simulink model "controller_v12"  (R2022a)
settings: Solver=FixedStepDiscrete  StartTime=0.0  StopTime=inf  RelTol=1e-3
undefined symbols (not defined in the file): ctr, DiscIntNeverNeededParam, flt, IO397, mdl, rbt, rsim, som, ukf_P0_flat, ukf_prediction_time, ukf_s0, ukf_sys, ukf_use_prediction
libraries: simulink x31, slrealtimeloglib x14, slrealtimetgmanagement x5, slrealtimeseriallib x5, speedgoatlib_fpga_analog_io x4, speedgoatlib_fpga x2, speedgoatlib_fpga_dio x1, slrealtimeutilitieslib x1
(part 2 of 4)

== system controller_v12/Force//Torque to Trajectory Specs/force//torque to module thrust ==
  note: No YAW torque control at the moment
  thrust : Inport
  x Tq : Inport  Port=2
  y Tq : Inport  Port=3
  z Tq : Inport  Port=4
  Inputs : slrealtimeloglib/File Log  Commented=on  decimation=1
      settings: SourceProductBaseCode=XP
  Mux : Mux
  SaturatingRamp : DiscreteIntegrator  gainval=1  SampleTime=-1  UpperSaturationLimit=1  LowerSaturationLimit=0  ICPrevOutput=DiscIntNeverNeededParam  ICPrevScaledInput=DiscIntNeverNeededParam
  constant : Constant
  mapping scheme (flipping compataible) : MATLAB Function  TreatAsAtomicUnit=on  SystemSampleTime=mdl.T
  module thrusts (1-4) : Outport  PortDimensions=4
  wires:
  thrust/1 -> Mux/1
  x Tq/1 -> Mux/2
  y Tq/1 -> Mux/3
  z Tq/1 -> Mux/4
  Mux/1 -> Inputs/1, mapping scheme (flipping compataible)/2(inputs)
  mapping scheme (flipping compataible)/1(module_f) -> module thrusts (1-4)/1
  constant/1 -> SaturatingRamp/1
  SaturatingRamp/1 -> mapping scheme (flipping compataible)/1(time)

== system controller_v12/Force//Torque to Trajectory Specs/nominal desired voltage ==
  Force : Inport
  Forces : slrealtimeloglib/File Log  Commented=on  decimation=1  inputProcessing=Elements as channels (sample based)
      settings: SourceProductBaseCode=XP
  SaturatingRamp : DiscreteIntegrator  gainval=1  SampleTime=-1  UpperSaturationLimit=1  LowerSaturationLimit=0  ICPrevOutput=DiscIntNeverNeededParam  ICPrevScaledInput=DiscIntNeverNeededParam
  Switch : Switch  Criteria=u2 > Threshold  SaturateOnIntegerOverflow=off  InputSameDT=off
  constant1 : Constant
  "force to voltage (hovering) " : Subsystem
  force to voltage flipping : Subsystem
  map_selection : MATLAB Function  TreatAsAtomicUnit=on  SystemSampleTime=mdl.T
  Voltages : Outport
  wires:
  Force/1 -> Forces/1, force to voltage flipping/1(force), "force to voltage (hovering) "/1(force)
  "force to voltage (hovering) "/1(Vout) -> Switch/1
  force to voltage flipping/1(Vout) -> Switch/3
  Switch/1 -> Voltages/1
  map_selection/1(hover_map) -> Switch/2
  constant1/1 -> SaturatingRamp/1
  SaturatingRamp/1 -> map_selection/1(time)

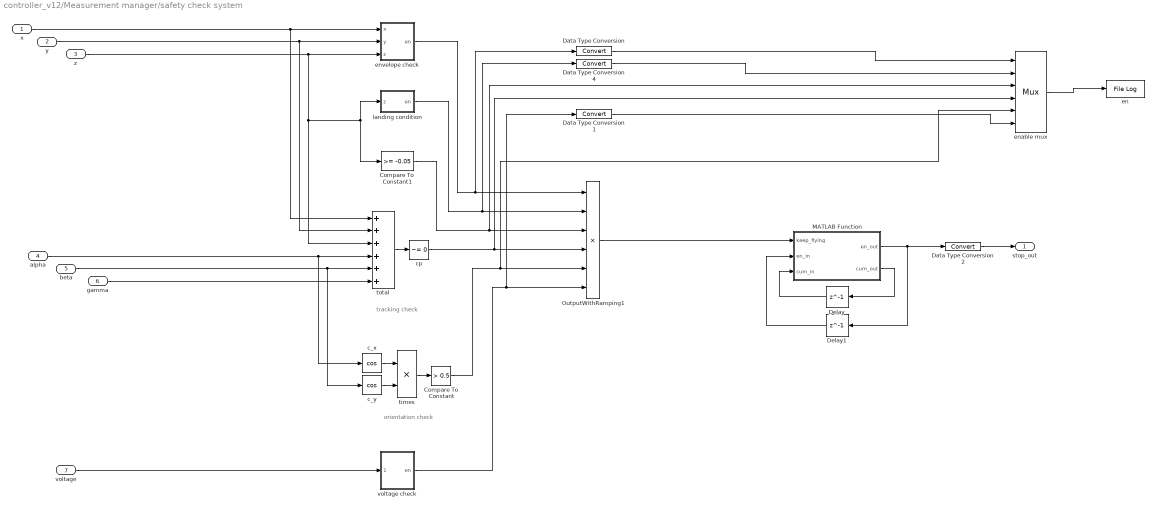
== system controller_v12/Measurement manager/safety check system ==
  note: orientation check
  note: tracking check
  x : Inport
  y : Inport  Port=2
  z : Inport  Port=3
  alpha : Inport  Port=4
  beta : Inport  Port=5
  gamma : Inport  Port=6
  voltage : Inport  Port=7
  Compare To Constant : simulink/Logic and Bit Operations/Compare To Constant  relop=>  const=0.5  OutDataTypeStr=uint8
  Compare To Constant1 : simulink/Logic and Bit Operations/Compare To Constant  relop=>=  const=-0.05  OutDataTypeStr=uint8
  Data Type Conversion{,1..2,4} (4 alike) : DataTypeConversion  SaturateOnIntegerOverflow=off  RndMeth=Floor
  Delay : Delay  DelayLength=1
  Delay1 : Delay  DelayLength=1  InitialCondition=1
  MATLAB Function : MATLAB Function  TreatAsAtomicUnit=on
  OutputWithRamping1 : Product  Inputs=6  RndMeth=Zero
  c_x : Trigonometry  Operator=cos
  c_y : Trigonometry  Operator=cos
  cp : simulink/Logic and Bit Operations/Compare To Zero  relop=~=  OutDataTypeStr=uint8
  en : slrealtimeloglib/File Log  decimation=1  inputProcessing=Elements as channels (sample based)
      settings: SourceProductBaseCode=XP
  enable mux : Mux  Inputs=6
      settings: DisplayOption=signals
  envelope check : MATLAB Function  TreatAsAtomicUnit=on
  landing condition : Subsystem
  times : Product  RndMeth=Zero
  total : Sum  Inputs=++++++
  voltage check : MATLAB Function  TreatAsAtomicUnit=on  SystemSampleTime=mdl.T
  stop_out : Outport
  wires:
  Compare To Constant1/1 -> enable mux/3, OutputWithRamping1/3
  y/1 -> envelope check/2(y), total/2
  cp/1 -> enable mux/4, OutputWithRamping1/4
  envelope check/1(en) -> Data Type Conversion/1, OutputWithRamping1/1
  enable mux/1 -> en/1
  landing condition/1(en) -> Data Type Conversion4/1, OutputWithRamping1/2
  Data Type Conversion/1 -> enable mux/1
  times/1 -> Compare To Constant/1
  voltage check/1(en) -> Data Type Conversion1/1, OutputWithRamping1/6
  z/1 -> total/3, Compare To Constant1/1, landing condition/1(z), envelope check/3(z)
  Compare To Constant/1 -> enable mux/5, OutputWithRamping1/5
  total/1 -> cp/1
  Data Type Conversion4/1 -> enable mux/2
  x/1 -> total/1, envelope check/1(x)
  alpha/1 -> total/4, c_x/1
  beta/1 -> total/5, c_y/1
  c_x/1 -> times/1
  c_y/1 -> times/2
  Data Type Conversion1/1 -> enable mux/6
  voltage/1 -> voltage check/1(voltage)
  gamma/1 -> total/6
  OutputWithRamping1/1 -> MATLAB Function/1(keep_flying)
  Delay1/1 -> MATLAB Function/2(en_in)
  MATLAB Function/1(en_out) -> Delay1/1, Data Type Conversion2/1
  Delay/1 -> MATLAB Function/3(cum_in)
  MATLAB Function/2(cum_out) -> Delay/1
  Data Type Conversion2/1 -> stop_out/1

== system controller_v12/Phantom trigger/timer1 ==
  SaturatingRamp : DiscreteIntegrator  gainval=1  SampleTime=-1  UpperSaturationLimit=1  LowerSaturationLimit=0  ICPrevOutput=DiscIntNeverNeededParam  ICPrevScaledInput=DiscIntNeverNeededParam
  constant : Constant
  time : Outport
  wires:
  constant/1 -> SaturatingRamp/1
  SaturatingRamp/1 -> time/1

== system controller_v12/closed loop en/safety1 ==
  In1 : Inport
  Compare To Constant1 : simulink/Logic and Bit Operations/Compare To Constant  relop=<=  const=inf  OutDataTypeStr=uint8
  Switch1 : Switch  Threshold=0.5  SaturateOnIntegerOverflow=off  InputSameDT=off
  zero1 : Constant  Value=0
  Out1 : Outport
  wires:
  In1/1 -> Switch1/1, Compare To Constant1/1
  Compare To Constant1/1 -> Switch1/2
  zero1/1 -> Switch1/3
  Switch1/1 -> Out1/1

== system controller_v12/closed loop en/safety2 ==
  In1 : Inport
  Compare To Constant1 : simulink/Logic and Bit Operations/Compare To Constant  relop=<=  const=inf  OutDataTypeStr=uint8
  Switch1 : Switch  Threshold=0.5  SaturateOnIntegerOverflow=off  InputSameDT=off
  zero1 : Constant  Value=0
  Out1 : Outport
  wires:
  In1/1 -> Switch1/1, Compare To Constant1/1
  Compare To Constant1/1 -> Switch1/2
  zero1/1 -> Switch1/3
  Switch1/1 -> Out1/1

== system controller_v12/closed loop en/safety3 ==
  In1 : Inport
  Compare To Constant1 : simulink/Logic and Bit Operations/Compare To Constant  relop=<=  const=inf  OutDataTypeStr=uint8
  Switch1 : Switch  Threshold=0.5  SaturateOnIntegerOverflow=off  InputSameDT=off
  zero1 : Constant  Value=0
  Out1 : Outport
  wires:
  In1/1 -> Switch1/1, Compare To Constant1/1
  Compare To Constant1/1 -> Switch1/2
  zero1/1 -> Switch1/3
  Switch1/1 -> Out1/1

== system controller_v12/closed loop en/safety4 ==
  In1 : Inport
  Compare To Constant1 : simulink/Logic and Bit Operations/Compare To Constant  relop=<=  const=inf  OutDataTypeStr=uint8
  Switch1 : Switch  Threshold=0.5  SaturateOnIntegerOverflow=off  InputSameDT=off
  zero1 : Constant  Value=0
  Out1 : Outport
  wires:
  In1/1 -> Switch1/1, Compare To Constant1/1
  Compare To Constant1/1 -> Switch1/2
  zero1/1 -> Switch1/3
  Switch1/1 -> Out1/1

== system controller_v12/signal generator/Bias_Signal ==
  note: time constant = 0.002sec
  QuasiEnable : Inport
  BiasVolts : Inport  Port=2
  AveragedBias : Subsystem
  PreGain : Gain
  Product : Product  RndMeth=Zero
  SIgnalForRamp_binary : Subsystem
  SaturatingRamp : DiscreteIntegrator  gainval=10  SampleTime=-1  LimitOutput=on  UpperSaturationLimit=1  LowerSaturationLimit=0  ICPrevOutput=DiscIntNeverNeededParam  ICPrevScaledInput=DiscIntNeverNeededParam
  BiasD2A : Outport
  wires:
  PreGain/1 -> BiasD2A/1
  BiasVolts/1 -> AveragedBias/1(In1)
  QuasiEnable/1 -> SIgnalForRamp_binary/1(In1)
  SIgnalForRamp_binary/1(Out1) -> SaturatingRamp/1
  SaturatingRamp/1 -> Product/1
  AveragedBias/1(Out1) -> Product/2
  Product/1 -> PreGain/1

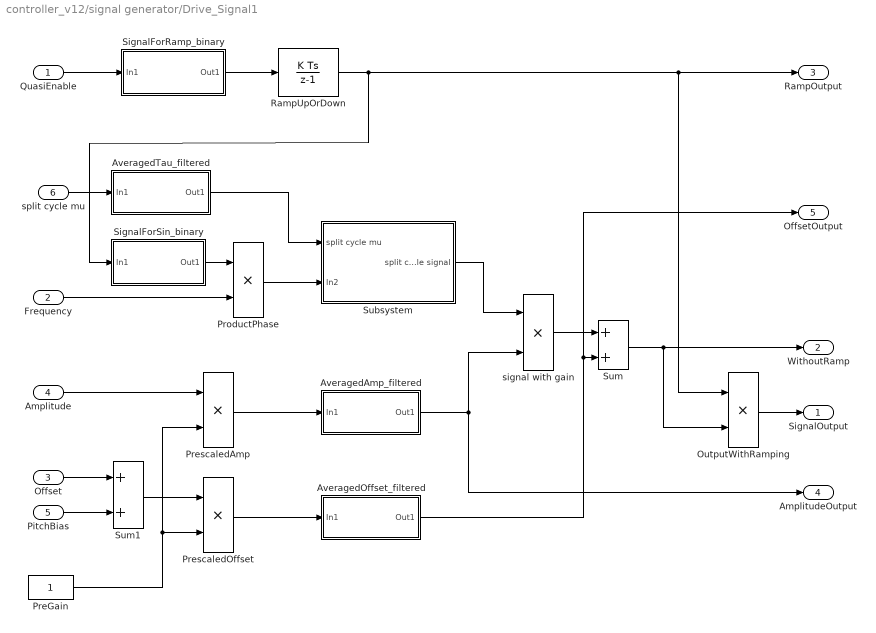
== system controller_v12/signal generator/Drive_Signal1 ==
  QuasiEnable : Inport
  Frequency : Inport  Port=2
  Offset : Inport  Port=3
  Amplitude : Inport  Port=4
  PitchBias : Inport  Port=5
  split cycle mu : Inport  Port=6
  AveragedAmp_filtered : Subsystem
  AveragedOffset_filtered : Subsystem
  AveragedTau_filtered : Subsystem
  OutputWithRamping : Product  RndMeth=Zero
  PreGain : Constant
  PrescaledAmp : Product  RndMeth=Zero
  PrescaledOffset : Product  RndMeth=Zero
  ProductPhase : Product  RndMeth=Zero
  RampUpOrDown : DiscreteIntegrator  gainval=10  SampleTime=-1  LimitOutput=on  UpperSaturationLimit=1  LowerSaturationLimit=0  ICPrevOutput=DiscIntNeverNeededParam  ICPrevScaledInput=DiscIntNeverNeededParam
  SignalForRamp_binary : Subsystem
  SignalForSin_binary : Subsystem
  Subsystem : Subsystem
  Sum : Sum
  Sum1 : Sum
  signal with gain : Product  RndMeth=Zero
  SignalOutput : Outport
  WithoutRamp : Outport  Port=2
  RampOutput : Outport  Port=3
  AmplitudeOutput : Outport  Port=4
  OffsetOutput : Outport  Port=5
  wires:
  PrescaledAmp/1 -> AveragedAmp_filtered/1(In1)
  Sum/1 -> OutputWithRamping/2, WithoutRamp/1
  RampUpOrDown/1 -> RampOutput/1, OutputWithRamping/1, SignalForSin_binary/1(In1)
  QuasiEnable/1 -> SignalForRamp_binary/1(In1)
  SignalForRamp_binary/1(Out1) -> RampUpOrDown/1
  Amplitude/1 -> PrescaledAmp/1
  signal with gain/1 -> Sum/1
  Frequency/1 -> ProductPhase/2
  SignalForSin_binary/1(Out1) -> ProductPhase/1
  ProductPhase/1 -> Subsystem/2(In2)
  AveragedOffset_filtered/1(Out1) -> Sum/2, OffsetOutput/1
  PrescaledOffset/1 -> AveragedOffset_filtered/1(In1)
  PreGain/1 -> PrescaledAmp/2, PrescaledOffset/2
  OutputWithRamping/1 -> SignalOutput/1
  AveragedAmp_filtered/1(Out1) -> signal with gain/2, AmplitudeOutput/1
  Sum1/1 -> PrescaledOffset/1
  Offset/1 -> Sum1/1
  PitchBias/1 -> Sum1/2
  AveragedTau_filtered/1(Out1) -> Subsystem/1(split cycle mu)
  split cycle mu/1 -> AveragedTau_filtered/1(In1)
  Subsystem/1(split cycle signal) -> signal with gain/1

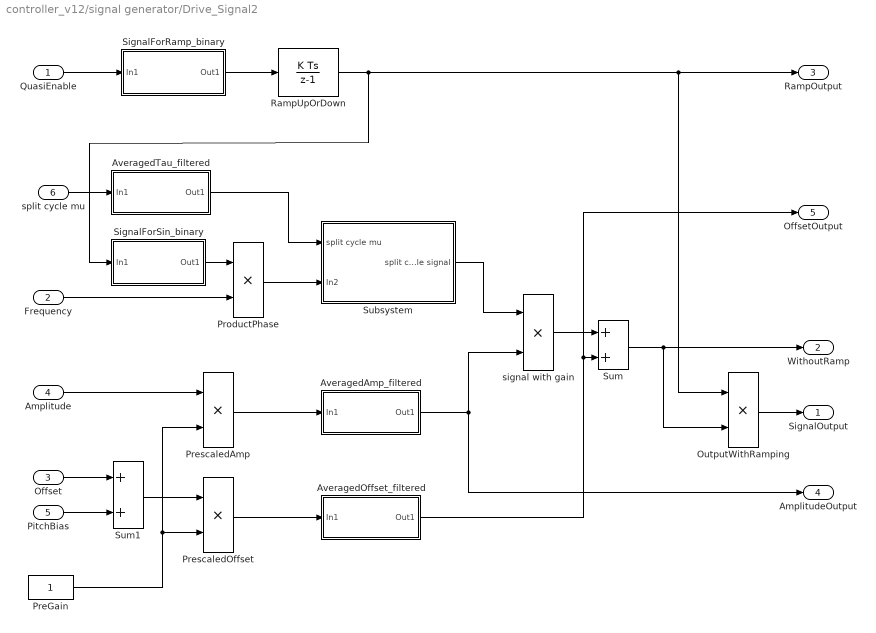
== system controller_v12/signal generator/Drive_Signal2 ==
  QuasiEnable : Inport
  Frequency : Inport  Port=2
  Offset : Inport  Port=3
  Amplitude : Inport  Port=4
  PitchBias : Inport  Port=5
  split cycle mu : Inport  Port=6
  AveragedAmp_filtered : Subsystem
  AveragedOffset_filtered : Subsystem
  AveragedTau_filtered : Subsystem
  OutputWithRamping : Product  RndMeth=Zero
  PreGain : Constant
  PrescaledAmp : Product  RndMeth=Zero
  PrescaledOffset : Product  RndMeth=Zero
  ProductPhase : Product  RndMeth=Zero
  RampUpOrDown : DiscreteIntegrator  gainval=10  SampleTime=-1  LimitOutput=on  UpperSaturationLimit=1  LowerSaturationLimit=0  ICPrevOutput=DiscIntNeverNeededParam  ICPrevScaledInput=DiscIntNeverNeededParam
  SignalForRamp_binary : Subsystem
  SignalForSin_binary : Subsystem
  Subsystem : Subsystem
  Sum : Sum
  Sum1 : Sum
  signal with gain : Product  RndMeth=Zero
  SignalOutput : Outport
  WithoutRamp : Outport  Port=2
  RampOutput : Outport  Port=3
  AmplitudeOutput : Outport  Port=4
  OffsetOutput : Outport  Port=5
  wires:
  PrescaledAmp/1 -> AveragedAmp_filtered/1(In1)
  Sum/1 -> OutputWithRamping/2, WithoutRamp/1
  RampUpOrDown/1 -> RampOutput/1, OutputWithRamping/1, SignalForSin_binary/1(In1)
  QuasiEnable/1 -> SignalForRamp_binary/1(In1)
  SignalForRamp_binary/1(Out1) -> RampUpOrDown/1
  Amplitude/1 -> PrescaledAmp/1
  signal with gain/1 -> Sum/1
  Frequency/1 -> ProductPhase/2
  SignalForSin_binary/1(Out1) -> ProductPhase/1
  ProductPhase/1 -> Subsystem/2(In2)
  AveragedOffset_filtered/1(Out1) -> Sum/2, OffsetOutput/1
  PrescaledOffset/1 -> AveragedOffset_filtered/1(In1)
  PreGain/1 -> PrescaledAmp/2, PrescaledOffset/2
  OutputWithRamping/1 -> SignalOutput/1
  AveragedAmp_filtered/1(Out1) -> signal with gain/2, AmplitudeOutput/1
  Sum1/1 -> PrescaledOffset/1
  Offset/1 -> Sum1/1
  PitchBias/1 -> Sum1/2
  AveragedTau_filtered/1(Out1) -> Subsystem/1(split cycle mu)
  split cycle mu/1 -> AveragedTau_filtered/1(In1)
  Subsystem/1(split cycle signal) -> signal with gain/1

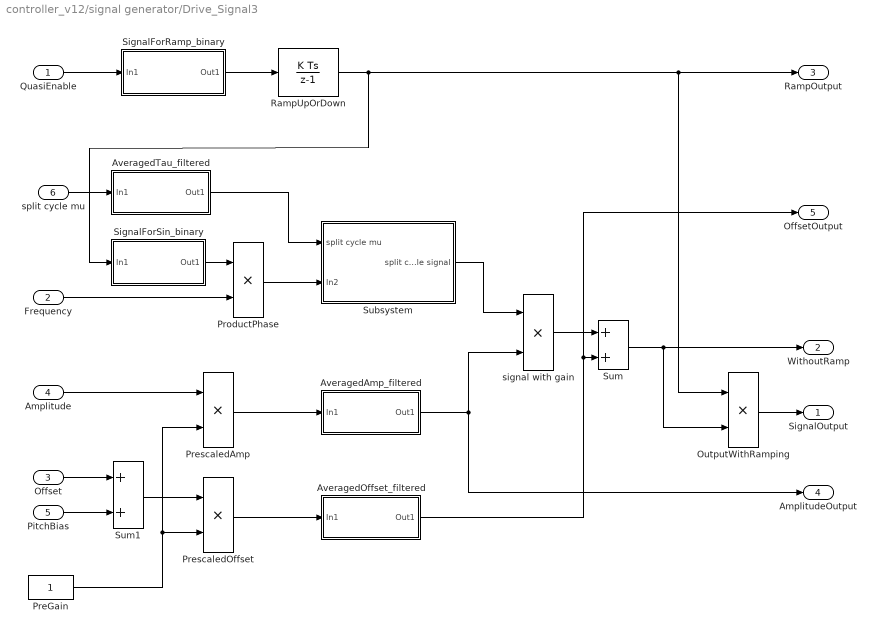
== system controller_v12/signal generator/Drive_Signal3 ==
  QuasiEnable : Inport
  Frequency : Inport  Port=2
  Offset : Inport  Port=3
  Amplitude : Inport  Port=4
  PitchBias : Inport  Port=5
  split cycle mu : Inport  Port=6
  AveragedAmp_filtered : Subsystem
  AveragedOffset_filtered : Subsystem
  AveragedTau_filtered : Subsystem
  OutputWithRamping : Product  RndMeth=Zero
  PreGain : Constant
  PrescaledAmp : Product  RndMeth=Zero
  PrescaledOffset : Product  RndMeth=Zero
  ProductPhase : Product  RndMeth=Zero
  RampUpOrDown : DiscreteIntegrator  gainval=10  SampleTime=-1  LimitOutput=on  UpperSaturationLimit=1  LowerSaturationLimit=0  ICPrevOutput=DiscIntNeverNeededParam  ICPrevScaledInput=DiscIntNeverNeededParam
  SignalForRamp_binary : Subsystem
  SignalForSin_binary : Subsystem
  Subsystem : Subsystem
  Sum : Sum
  Sum1 : Sum
  signal with gain : Product  RndMeth=Zero
  SignalOutput : Outport
  WithoutRamp : Outport  Port=2
  RampOutput : Outport  Port=3
  AmplitudeOutput : Outport  Port=4
  OffsetOutput : Outport  Port=5
  wires:
  PrescaledAmp/1 -> AveragedAmp_filtered/1(In1)
  Sum/1 -> OutputWithRamping/2, WithoutRamp/1
  RampUpOrDown/1 -> RampOutput/1, OutputWithRamping/1, SignalForSin_binary/1(In1)
  QuasiEnable/1 -> SignalForRamp_binary/1(In1)
  SignalForRamp_binary/1(Out1) -> RampUpOrDown/1
  Amplitude/1 -> PrescaledAmp/1
  signal with gain/1 -> Sum/1
  Frequency/1 -> ProductPhase/2
  SignalForSin_binary/1(Out1) -> ProductPhase/1
  ProductPhase/1 -> Subsystem/2(In2)
  AveragedOffset_filtered/1(Out1) -> Sum/2, OffsetOutput/1
  PrescaledOffset/1 -> AveragedOffset_filtered/1(In1)
  PreGain/1 -> PrescaledAmp/2, PrescaledOffset/2
  OutputWithRamping/1 -> SignalOutput/1
  AveragedAmp_filtered/1(Out1) -> signal with gain/2, AmplitudeOutput/1
  Sum1/1 -> PrescaledOffset/1
  Offset/1 -> Sum1/1
  PitchBias/1 -> Sum1/2
  AveragedTau_filtered/1(Out1) -> Subsystem/1(split cycle mu)
  split cycle mu/1 -> AveragedTau_filtered/1(In1)
  Subsystem/1(split cycle signal) -> signal with gain/1

== system controller_v12/signal generator/Drive_Signal4 ==
  QuasiEnable : Inport
  Frequency : Inport  Port=2
  Offset : Inport  Port=3
  Amplitude : Inport  Port=4
  PitchBias : Inport  Port=5
  split cycle mu : Inport  Port=6
  AveragedAmp_filtered : Subsystem
  AveragedOffset_filtered : Subsystem
  AveragedTau_filtered : Subsystem
  OutputWithRamping : Product  RndMeth=Zero
  PreGain : Constant
  PrescaledAmp : Product  RndMeth=Zero
  PrescaledOffset : Product  RndMeth=Zero
  ProductPhase : Product  RndMeth=Zero
  RampUpOrDown : DiscreteIntegrator  gainval=10  SampleTime=-1  LimitOutput=on  UpperSaturationLimit=1  LowerSaturationLimit=0  ICPrevOutput=DiscIntNeverNeededParam  ICPrevScaledInput=DiscIntNeverNeededParam
  SignalForRamp_binary : Subsystem
  SignalForSin_binary : Subsystem
  Subsystem : Subsystem
  Sum : Sum
  Sum1 : Sum
  signal with gain : Product  RndMeth=Zero
  SignalOutput : Outport
  WithoutRamp : Outport  Port=2
  RampOutput : Outport  Port=3
  AmplitudeOutput : Outport  Port=4
  OffsetOutput : Outport  Port=5
  wires:
  PrescaledAmp/1 -> AveragedAmp_filtered/1(In1)
  Sum/1 -> OutputWithRamping/2, WithoutRamp/1
  RampUpOrDown/1 -> RampOutput/1, OutputWithRamping/1, SignalForSin_binary/1(In1)
  QuasiEnable/1 -> SignalForRamp_binary/1(In1)
  SignalForRamp_binary/1(Out1) -> RampUpOrDown/1
  Amplitude/1 -> PrescaledAmp/1
  signal with gain/1 -> Sum/1
  Frequency/1 -> ProductPhase/2
  SignalForSin_binary/1(Out1) -> ProductPhase/1
  ProductPhase/1 -> Subsystem/2(In2)
  AveragedOffset_filtered/1(Out1) -> Sum/2, OffsetOutput/1
  PrescaledOffset/1 -> AveragedOffset_filtered/1(In1)
  PreGain/1 -> PrescaledAmp/2, PrescaledOffset/2
  OutputWithRamping/1 -> SignalOutput/1
  AveragedAmp_filtered/1(Out1) -> signal with gain/2, AmplitudeOutput/1
  Sum1/1 -> PrescaledOffset/1
  Offset/1 -> Sum1/1
  PitchBias/1 -> Sum1/2
  AveragedTau_filtered/1(Out1) -> Subsystem/1(split cycle mu)
  split cycle mu/1 -> AveragedTau_filtered/1(In1)
  Subsystem/1(split cycle signal) -> signal with gain/1

== system controller_v12/signal generator/SignalSaturationLimit ==
  BiasMax : Inport
  SignalRaw : Inport  Port=2
  GainBias : Gain
  MaxOf : MinMax  Function=max  Inputs=2
  MinOf : MinMax  Inputs=2
  ground : Constant
  SignalSatd : Outport
  wires:
  BiasMax/1 -> GainBias/1
  SignalRaw/1 -> MinOf/2
  MinOf/1 -> MaxOf/1
  MaxOf/1 -> SignalSatd/1
  GainBias/1 -> MinOf/1
  ground/1 -> MaxOf/2

== system controller_v12/signal generator/SignalSaturationLimit1 ==
  BiasMax : Inport
  SignalRaw : Inport  Port=2
  GainBias : Gain
  MaxOf : MinMax  Function=max  Inputs=2
  MinOf : MinMax  Inputs=2
  ground : Constant
  SignalSatd : Outport
  wires:
  BiasMax/1 -> GainBias/1
  SignalRaw/1 -> MinOf/2
  MinOf/1 -> MaxOf/1
  MaxOf/1 -> SignalSatd/1
  GainBias/1 -> MinOf/1
  ground/1 -> MaxOf/2

== system controller_v12/signal generator/SignalSaturationLimit2 ==
  BiasMax : Inport
  SignalRaw : Inport  Port=2
  GainBias : Gain
  MaxOf : MinMax  Function=max  Inputs=2
  MinOf : MinMax  Inputs=2
  ground : Constant
  SignalSatd : Outport
  wires:
  BiasMax/1 -> GainBias/1
  SignalRaw/1 -> MinOf/2
  MinOf/1 -> MaxOf/1
  MaxOf/1 -> SignalSatd/1
  GainBias/1 -> MinOf/1
  ground/1 -> MaxOf/2

== system controller_v12/signal generator/SignalSaturationLimit3 ==
  BiasMax : Inport
  SignalRaw : Inport  Port=2
  GainBias : Gain
  MaxOf : MinMax  Function=max  Inputs=2
  MinOf : MinMax  Inputs=2
  ground : Constant
  SignalSatd : Outport
  wires:
  BiasMax/1 -> GainBias/1
  SignalRaw/1 -> MinOf/2
  MinOf/1 -> MaxOf/1
  MaxOf/1 -> SignalSatd/1
  GainBias/1 -> MinOf/1
  ground/1 -> MaxOf/2

== system controller_v12/Adaptive Controller/adaptive system/integrator ==
  note: integrator limit (saturation) needs to be set.
  e : Inport
  torque offset : Inport  Port=2
  thrust_offset : Inport  Port=3
  enable1 : Product  Inputs=**
  initial guess : MATLAB Function  TreatAsAtomicUnit=on
  integrator with sat : DiscreteIntegrator  IntegratorMethod=Integration: Backward Euler  gainval=1  SampleTime=-1  LimitOutput=on  UpperSaturationLimit=ctr.integral.lim.upper  LowerSaturationLimit=ctr.integral.lim.lower  ICPrevOutput=DiscIntNeverNeededParam  ICPrevScaledInput=DiscIntNeverNeededParam
  safety2 : Subsystem
  start ramp : Subsystem
  int_e : Outport
  " torq_off" : Outport  Port=2
  th_off : Outport  Port=3
  wires:
  safety2/1(Out1) -> enable1/2
  enable1/1 -> integrator with sat/1
  start ramp/1(Out1) -> enable1/1
  e/1 -> safety2/1(In1)
  integrator with sat/1 -> initial guess/1(i_e)
  initial guess/1(int_e) -> int_e/1
  initial guess/2(tor_inte) -> " torq_off"/1
  initial guess/3(th_inte) -> th_off/1
  torque offset/1 -> initial guess/2(tor_off)
  thrust_offset/1 -> initial guess/3(th_off)

== system controller_v12/Adaptive Controller/adaptive system/safety1 ==
  In1 : Inport
  Compare To Constant1 : simulink/Logic and Bit Operations/Compare To Constant  relop=<=  const=inf  OutDataTypeStr=uint8
  Switch1 : Switch  Threshold=0.5  SaturateOnIntegerOverflow=off  InputSameDT=off
  zero1 : Constant  Value=0
  Out1 : Outport
  wires:
  In1/1 -> Switch1/1, Compare To Constant1/1
  Compare To Constant1/1 -> Switch1/2
  zero1/1 -> Switch1/3
  Switch1/1 -> Out1/1

== system controller_v12/Adaptive Controller/adaptive system/safety2 ==
  In1 : Inport
  Compare To Constant1 : simulink/Logic and Bit Operations/Compare To Constant  relop=<=  const=inf  OutDataTypeStr=uint8
  Switch1 : Switch  Threshold=0.5  SaturateOnIntegerOverflow=off  InputSameDT=off
  zero1 : Constant  Value=0
  Out1 : Outport
  wires:
  In1/1 -> Switch1/1, Compare To Constant1/1
  Compare To Constant1/1 -> Switch1/2
  zero1/1 -> Switch1/3
  Switch1/1 -> Out1/1

== system controller_v12/Adaptive Controller/attitude and thrust MPC controller/time ==
  constant : Constant
  time : DiscreteIntegrator  gainval=1  SampleTime=-1  UpperSaturationLimit=1  LowerSaturationLimit=0  ICPrevOutput=DiscIntNeverNeededParam  ICPrevScaledInput=DiscIntNeverNeededParam
  real times : Outport
  wires:
  constant/1 -> time/1
  time/1 -> real times/1

== system controller_v12/Adaptive Controller/attitude and thrust MPC controller2/NN RTMPC ==
  time : Inport
  r : Inport  Port=2
  r_dot : Inport  Port=3
  r_dotdot : Inport  Port=4
  R : Inport  Port=5
  Omega : Inport  Port=6
  rd : Inport  Port=7
  rd_d : Inport  Port=8
  rd_dd : Inport  Port=9
  rd_ddd : Inport  Port=10
  rd_dddd : Inport  Port=11
  int_e : Inport  Port=12
  MATLAB Function : MATLAB Function  TreatAsAtomicUnit=on
  MATLAB Function1 : MATLAB Function  TreatAsAtomicUnit=on
  MATLAB Function2 : MATLAB Function  TreatAsAtomicUnit=on
  Normalize NN Inputs : Gain  Gain=1/10
  Normalize NN Outputs : Gain  Gain=12
  Rd : Outport
  Omegad : Outport  Port=2
  cmd_B_acc_z : Outport  Port=3
  alt_e : Outport  Port=4
  wires:
  MATLAB Function1/1(Rd) -> Rd/1
  rd/1 -> MATLAB Function/7(rd)
  MATLAB Function1/4(alt_e) -> alt_e/1
  MATLAB Function1/2(Omegad) -> Omegad/1
  rd_d/1 -> MATLAB Function/8(rd_d)
  rd_dddd/1 -> MATLAB Function/11(rd_dddd)
  MATLAB Function1/3(cmd_B_acc_z) -> cmd_B_acc_z/1
  r_dotdot/1 -> MATLAB Function/4(r_dotdot)
  r_dot/1 -> MATLAB Function/3(r_dot)
  MATLAB Function/1(x_in) -> Normalize NN Inputs/1
  int_e/1 -> MATLAB Function/12(int_e)
  time/1 -> MATLAB Function/1(time)
  rd_dd/1 -> MATLAB Function/9(rd_dd)
  rd_ddd/1 -> MATLAB Function/10(rd_ddd)
  Omega/1 -> MATLAB Function/6(Omega)
  r/1 -> MATLAB Function/2(r)
  R/1 -> MATLAB Function1/2(R), MATLAB Function/5(R)
  Normalize NN Inputs/1 -> MATLAB Function2/1(x)
  Normalize NN Outputs/1 -> MATLAB Function1/1(u_nn)
  MATLAB Function2/1(y) -> Normalize NN Outputs/1

== system controller_v12/Adaptive Controller/attitude and thrust MPC controller2/time ==
  constant : Constant
  time : DiscreteIntegrator  gainval=1  SampleTime=-1  UpperSaturationLimit=1  LowerSaturationLimit=0  ICPrevOutput=DiscIntNeverNeededParam  ICPrevScaledInput=DiscIntNeverNeededParam
  real times : Outport
  wires:
  constant/1 -> time/1
  time/1 -> real times/1

== system controller_v12/Adaptive Controller/observer/ICRA'23 ==
  XYZ : Inport
  f_cmd : Inport  Port=2
  Euler : Inport  Port=3
  Rotaion : Subsystem
  Terminator : Terminator
  Terminator1 : Terminator
  Terminator2 : Terminator
  lateral KF observer : Subsystem
  lateral observer : Subsystem  Commented=on
  r : Outport
  r_dot : Outport  Port=2
  r_dotdot : Outport  Port=3
  R : Outport  Port=4
  Rdot : Outport  Port=5
  Omega : Outport  Port=6
  wires:
  Rotaion/2(Rdot) -> Rdot/1
  lateral observer/1(r) -> Terminator/1
  Rotaion/1(R) -> R/1, lateral KF observer/1(R)
  Rotaion/3(Omega) -> Omega/1
  lateral observer/2(r_dot) -> Terminator1/1
  XYZ/1 -> lateral KF observer/3(xyz), lateral observer/1(XYZ)
  lateral KF observer/1(r) -> r/1
  lateral KF observer/2(r_dot) -> r_dot/1
  f_cmd/1 -> lateral KF observer/2(f_cmd)
  lateral observer/3(r_dotdot) -> Terminator2/1
  Euler/1 -> Rotaion/1(Euler)
  lateral KF observer/3(r_dotdot) -> r_dotdot/1

== system controller_v12/Adaptive Controller/observer/observer ==
  xyz : Inport
  euler : Inport  Port=2
  f_cmd : Inport  Port=3
  tau_cmd_x : Inport  Port=4
  tau_cmd_y : Inport  Port=5
  Constant : Constant  Value=zeros(3,1)
  Constant1 : Constant  Value=zeros(9,1)
  Mux : Mux
  Overload Options : slrealtimetgmanagement/Overload Options  startupDur=10  startupDurSrc=Tunable Parameter  maxOverload=10  maxOverloadSrc=Tunable Parameter  TETFlag=on
      settings: SourceProductBaseCode=XP
  Terminator1 : Terminator  Commented=on
  Terminator2 : Terminator  Commented=on
  To Workspace3 : ToWorkspace  VariableName=ukf_r_out  SaveFormat=Timeseries  SampleTime=-1
  To Workspace4 : ToWorkspace  VariableName=ukf_r_dot_out  SaveFormat=Timeseries  SampleTime=-1
  To Workspace5 : ToWorkspace  VariableName=ukf_R_out  SaveFormat=Timeseries  SampleTime=-1
  To Workspace6 : ToWorkspace  VariableName=ukf_omega_out  SaveFormat=Timeseries  SampleTime=-1
  UKF : Subsystem
  UKF1 : Subsystem
  lateral observer : Subsystem  Commented=on
  ukf_prediction_time : Constant  Value=ukf_prediction_time
  r : Outport
  r_dot : Outport  Port=2
  r_dotdot : Outport  Port=3
  R : Outport  Port=4
  Omega : Outport  Port=5
  Rdot : Outport  Port=6
  wires:
  euler/1 -> UKF/2(euler)
  xyz/1 -> UKF/1(r_in)
  f_cmd/1 -> UKF/5(f_cmd)
  tau_cmd_x/1 -> UKF/6(tau_cmd_x)
  tau_cmd_y/1 -> UKF/7(tau_cmd_y)
  UKF/4(omega_out) -> Mux/4, To Workspace6/1, Omega/1
  UKF/3(R_out) -> Mux/3, R/1, To Workspace5/1
  UKF/2(r_dot_out) -> Mux/2, r_dot/1, To Workspace4/1
  UKF/1(r_out) -> Mux/1, To Workspace3/1, r/1
  Constant/1 -> r_dotdot/1, UKF/4(omega_in), UKF/3(r_dot_in)
  Constant1/1 -> Rdot/1
  Overload Options/2 -> Terminator1/1  "UKF TET"
  Overload Options/1 -> Terminator2/1  "UKF count"
  Mux/1 -> Overload Options/1
  ukf_prediction_time/1 -> ?

== system controller_v12/Force//Torque to Trajectory Specs/nominal desired voltage/force to voltage (hovering)  ==
  note: apply max voltage limit
  note: known correction from open-loop tests
  force : Inport
  Add : Sum  Inputs=+++
  Constant : Constant  Value=rbt.VM_input1
  Constant1 : Constant  Value=rbt.DV
  Constant2 : Constant  Value=rbt.VM_input2
  MATLAB Function : MATLAB Function  TreatAsAtomicUnit=on
  Product : Product
  Vout : Outport
  wires:
  MATLAB Function/1(Vo) -> Vout/1
  force/1 -> Product/2
  Constant2/1 -> Add/2
  Product/1 -> Add/3
  Add/1 -> MATLAB Function/1(Vi)
  Constant1/1 -> Add/1
  Constant/1 -> Product/1

== system controller_v12/Force//Torque to Trajectory Specs/nominal desired voltage/force to voltage flipping ==
  note: apply max voltage limit
  note: known correction from open-loop tests
  force : Inport
  Add : Sum
  Constant : Constant  Value=rbt.VM2
  Constant1 : Constant  Value=rbt.DV_flip
  MATLAB Function : MATLAB Function  TreatAsAtomicUnit=on
  Product : Product
  Sqrt : Sqrt
  Vout : Outport
  wires:
  MATLAB Function/1(Vo) -> Vout/1
  force/1 -> Sqrt/1
  Add/1 -> MATLAB Function/1(Vi)
  Constant1/1 -> Add/1
  Constant/1 -> Product/1
  Product/1 -> Add/2
  Sqrt/1 -> Product/2

== system controller_v12/Measurement manager/safety check system/landing condition ==
  z : Inport
  Add : Sum  Inputs=+--
  SaturatingRamp1 : DiscreteIntegrator  gainval=1  SampleTime=-1  UpperSaturationLimit=1  LowerSaturationLimit=0  ICPrevOutput=DiscIntNeverNeededParam  ICPrevScaledInput=DiscIntNeverNeededParam
  constant : Constant
  constant1 : Constant  Value=2
  constant2 : Constant  Value=mdl.i_delay
  landing_cond : MATLAB Function  TreatAsAtomicUnit=on  SystemSampleTime=mdl.T
  en : Outport
  wires:
  SaturatingRamp1/1 -> Add/1
  constant/1 -> SaturatingRamp1/1
  constant1/1 -> Add/2
  constant2/1 -> Add/3
  Add/1 -> landing_cond/2(time_cond)
  z/1 -> landing_cond/1(alt)
  landing_cond/1(en) -> en/1

== system controller_v12/signal generator/Bias_Signal/AveragedBias ==
  note: To avoid having signal "jump",
      | we want SMOOTH transitions
      | in frequency (i.e., a weighted sum
      | of current freq and freq some delta t ago)
  note: time constant = 0.002sec
  In1 : Inport
  Discrete Transfer Fcn : DiscreteTransferFcn  Numerator=[0.05]  Denominator=[1 -.95]
  Out1 : Outport
  wires:
  In1/1 -> Discrete Transfer Fcn/1
  Discrete Transfer Fcn/1 -> Out1/1

== system controller_v12/signal generator/Bias_Signal/SIgnalForRamp_binary ==
  note: Should output 1 or -1,
      | so signal ramps UP to 1
      | or DOWN to 0.
  In1 : Inport
  Add : Sum  Inputs=+-
  Compare To Zero : simulink/Logic and Bit Operations/Compare To Zero  relop=>  OutDataTypeStr=uint8  ZeroCross=off
  Constant : Constant
  Data Type Conversion : DataTypeConversion  OutDataTypeStr=double  SaturateOnIntegerOverflow=off  RndMeth=Floor
  Gain : Gain  Gain=2
  Out1 : Outport
  wires:
  In1/1 -> Compare To Zero/1
  Compare To Zero/1 -> Data Type Conversion/1
  Gain/1 -> Add/1
  Constant/1 -> Add/2
  Add/1 -> Out1/1
  Data Type Conversion/1 -> Gain/1

== system controller_v12/signal generator/Drive_Signal1/AveragedAmp_filtered ==
  note: To avoid having signal "jump",
      | we want SMOOTH transitions
      | in frequency (i.e., a weighted sum
      | of current freq and freq some delta t ago)
  note: time constant 0.002sec
      | for 10kHz samping
  In1 : Inport
  Discrete Transfer Fcn : DiscreteTransferFcn  Numerator=[0.05]  Denominator=[1 -.95]
  Out1 : Outport
  wires:
  In1/1 -> Discrete Transfer Fcn/1
  Discrete Transfer Fcn/1 -> Out1/1

== system controller_v12/signal generator/Drive_Signal1/AveragedOffset_filtered ==
  note: To avoid having signal "jump",
      | we want SMOOTH transitions
      | in frequency (i.e., a weighted sum
      | of current freq and freq some delta t ago)
  note: c
  note: time constant 0.02sec
      | for 10kHz samping
  In1 : Inport
  Discrete Transfer Fcn : DiscreteTransferFcn  Numerator=[0.05]  Denominator=[1 -.95]
  Out1 : Outport
  wires:
  In1/1 -> Discrete Transfer Fcn/1
  Discrete Transfer Fcn/1 -> Out1/1

== system controller_v12/signal generator/Drive_Signal1/AveragedTau_filtered ==
  note: To avoid having signal "jump",
      | we want SMOOTH transitions
      | in frequency (i.e., a weighted sum
      | of current freq and freq some delta t ago)
  note: time constant 0.002sec
      | for 10kHz samping
  In1 : Inport
  Discrete Transfer Fcn : DiscreteTransferFcn  Numerator=[0.05]  Denominator=[1, -0.95]
  Out1 : Outport
  wires:
  In1/1 -> Discrete Transfer Fcn/1
  Discrete Transfer Fcn/1 -> Out1/1

== system controller_v12/signal generator/Drive_Signal1/SignalForRamp_binary ==
  note: Should output 1 or -1,
      | so signal ramps UP to 1
      | or DOWN to 0.
  In1 : Inport
  Add : Sum  Inputs=+-
  Compare To Zero : simulink/Logic and Bit Operations/Compare To Zero  relop=>  OutDataTypeStr=uint8  ZeroCross=off
  Constant : Constant
  Data Type Conversion : DataTypeConversion  OutDataTypeStr=double  SaturateOnIntegerOverflow=off  RndMeth=Floor
  Gain : Gain  Gain=2
  Out1 : Outport
  wires:
  In1/1 -> Compare To Zero/1
  Compare To Zero/1 -> Data Type Conversion/1
  Gain/1 -> Add/1
  Constant/1 -> Add/2
  Add/1 -> Out1/1
  Data Type Conversion/1 -> Gain/1

== system controller_v12/signal generator/Drive_Signal1/SignalForSin_binary ==
  note: We want this to stay "high" for 1
      | second after the actual "enable"
      | is turned off...
  In1 : Inport
  Compare To Zero : simulink/Logic and Bit Operations/Compare To Zero  relop=>  OutDataTypeStr=uint8  ZeroCross=off
  Data Type Conversion : DataTypeConversion  OutDataTypeStr=double  SaturateOnIntegerOverflow=off  RndMeth=Floor
  Out1 : Outport
  wires:
  In1/1 -> Compare To Zero/1
  Compare To Zero/1 -> Data Type Conversion/1
  Data Type Conversion/1 -> Out1/1

== system controller_v12/signal generator/Drive_Signal1/Subsystem ==
  note: positive value pushes the left wing forward
  split cycle mu : Inport
  In2 : Inport  Port=2
  1-mu : Sum  Inputs=+-
  2f : Gain  Gain=2
  2nd harmonic : Trigonometry  OutputSignalType=real
  2pi : Gain  Gain=2*pi
  Abs1 : Abs  SaturateOnIntegerOverflow=off
  Add : Sum
  Constant : Constant
  combined sines : Sum
  deg to rad : Gain  Gain=pi/180
  f : Gain  Gain=-1
  first harmonic : Trigonometry  OutputSignalType=real
  omega*t : DiscreteIntegrator  SampleTime=-1  ICPrevOutput=DiscIntNeverNeededParam  ICPrevScaledInput=DiscIntNeverNeededParam
  phase offset : Constant  Value=0
  signal with gain1 : Product  RndMeth=Zero
  signal with gain2 : Product  RndMeth=Zero
  split cycle signal : Outport
  wires:
  2f/1 -> 2nd harmonic/1
  first harmonic/1 -> signal with gain1/2
  Constant/1 -> 1-mu/1
  split cycle mu/1 -> f/1, Abs1/1
  1-mu/1 -> signal with gain1/1
  2nd harmonic/1 -> signal with gain2/2
  signal with gain1/1 -> combined sines/1
  signal with gain2/1 -> combined sines/2
  combined sines/1 -> split cycle signal/1
  f/1 -> signal with gain2/1
  Abs1/1 -> 1-mu/2
  In2/1 -> 2pi/1
  2pi/1 -> omega*t/1
  omega*t/1 -> Add/2
  Add/1 -> first harmonic/1, 2f/1
  phase offset/1 -> deg to rad/1
  deg to rad/1 -> Add/1

== system controller_v12/signal generator/Drive_Signal2/AveragedAmp_filtered ==
  note: To avoid having signal "jump",
      | we want SMOOTH transitions
      | in frequency (i.e., a weighted sum
      | of current freq and freq some delta t ago)
  note: time constant 0.002sec
      | for 10kHz samping
  In1 : Inport
  Discrete Transfer Fcn : DiscreteTransferFcn  Numerator=[0.05]  Denominator=[1 -.95]
  Out1 : Outport
  wires:
  In1/1 -> Discrete Transfer Fcn/1
  Discrete Transfer Fcn/1 -> Out1/1

== system controller_v12/signal generator/Drive_Signal2/AveragedOffset_filtered ==
  note: To avoid having signal "jump",
      | we want SMOOTH transitions
      | in frequency (i.e., a weighted sum
      | of current freq and freq some delta t ago)
  note: c
  note: time constant 0.02sec
      | for 10kHz samping
  In1 : Inport
  Discrete Transfer Fcn : DiscreteTransferFcn  Numerator=[0.05]  Denominator=[1 -.95]
  Out1 : Outport
  wires:
  In1/1 -> Discrete Transfer Fcn/1
  Discrete Transfer Fcn/1 -> Out1/1

== system controller_v12/signal generator/Drive_Signal2/AveragedTau_filtered ==
  note: To avoid having signal "jump",
      | we want SMOOTH transitions
      | in frequency (i.e., a weighted sum
      | of current freq and freq some delta t ago)
  note: time constant 0.002sec
      | for 10kHz samping
  In1 : Inport
  Discrete Transfer Fcn : DiscreteTransferFcn  Numerator=[0.05]  Denominator=[1, -0.95]
  Out1 : Outport
  wires:
  In1/1 -> Discrete Transfer Fcn/1
  Discrete Transfer Fcn/1 -> Out1/1

== system controller_v12/signal generator/Drive_Signal2/SignalForRamp_binary ==
  note: Should output 1 or -1,
      | so signal ramps UP to 1
      | or DOWN to 0.
  In1 : Inport
  Add : Sum  Inputs=+-
  Compare To Zero : simulink/Logic and Bit Operations/Compare To Zero  relop=>  OutDataTypeStr=uint8  ZeroCross=off
  Constant : Constant
  Data Type Conversion : DataTypeConversion  OutDataTypeStr=double  SaturateOnIntegerOverflow=off  RndMeth=Floor
  Gain : Gain  Gain=2
  Out1 : Outport
  wires:
  In1/1 -> Compare To Zero/1
  Compare To Zero/1 -> Data Type Conversion/1
  Gain/1 -> Add/1
  Constant/1 -> Add/2
  Add/1 -> Out1/1
  Data Type Conversion/1 -> Gain/1

== system controller_v12/signal generator/Drive_Signal2/SignalForSin_binary ==
  note: We want this to stay "high" for 1
      | second after the actual "enable"
      | is turned off...
  In1 : Inport
  Compare To Zero : simulink/Logic and Bit Operations/Compare To Zero  relop=>  OutDataTypeStr=uint8  ZeroCross=off
  Data Type Conversion : DataTypeConversion  OutDataTypeStr=double  SaturateOnIntegerOverflow=off  RndMeth=Floor
  Out1 : Outport
  wires:
  In1/1 -> Compare To Zero/1
  Compare To Zero/1 -> Data Type Conversion/1
  Data Type Conversion/1 -> Out1/1

== system controller_v12/signal generator/Drive_Signal2/Subsystem ==
  note: positive value pushes the left wing forward
  split cycle mu : Inport
  In2 : Inport  Port=2
  1-mu : Sum  Inputs=+-
  2f : Gain  Gain=2
  2nd harmonic : Trigonometry  OutputSignalType=real
  2pi : Gain  Gain=2*pi
  Abs1 : Abs  SaturateOnIntegerOverflow=off
  Add : Sum
  Constant : Constant
  combined sines : Sum
  deg to rad : Gain  Gain=pi/180
  f : Gain  Gain=-1
  first harmonic : Trigonometry  OutputSignalType=real
  omega*t : DiscreteIntegrator  SampleTime=-1  ICPrevOutput=DiscIntNeverNeededParam  ICPrevScaledInput=DiscIntNeverNeededParam
  phase offset : Constant  Value=180
  signal with gain1 : Product  RndMeth=Zero
  signal with gain2 : Product  RndMeth=Zero
  split cycle signal : Outport
  wires:
  2f/1 -> 2nd harmonic/1
  first harmonic/1 -> signal with gain1/2
  Constant/1 -> 1-mu/1
  split cycle mu/1 -> f/1, Abs1/1
  1-mu/1 -> signal with gain1/1
  2nd harmonic/1 -> signal with gain2/2
  signal with gain1/1 -> combined sines/1
  signal with gain2/1 -> combined sines/2
  combined sines/1 -> split cycle signal/1
  f/1 -> signal with gain2/1
  Abs1/1 -> 1-mu/2
  In2/1 -> 2pi/1
  2pi/1 -> omega*t/1
  omega*t/1 -> Add/2
  Add/1 -> first harmonic/1, 2f/1
  phase offset/1 -> deg to rad/1
  deg to rad/1 -> Add/1

== system controller_v12/signal generator/Drive_Signal3/AveragedAmp_filtered ==
  note: To avoid having signal "jump",
      | we want SMOOTH transitions
      | in frequency (i.e., a weighted sum
      | of current freq and freq some delta t ago)
  note: time constant 0.002sec
      | for 10kHz samping
  In1 : Inport
  Discrete Transfer Fcn : DiscreteTransferFcn  Numerator=[0.05]  Denominator=[1 -.95]
  Out1 : Outport
  wires:
  In1/1 -> Discrete Transfer Fcn/1
  Discrete Transfer Fcn/1 -> Out1/1

== system controller_v12/signal generator/Drive_Signal3/AveragedOffset_filtered ==
  note: To avoid having signal "jump",
      | we want SMOOTH transitions
      | in frequency (i.e., a weighted sum
      | of current freq and freq some delta t ago)
  note: c
  note: time constant 0.02sec
      | for 10kHz samping
  In1 : Inport
  Discrete Transfer Fcn : DiscreteTransferFcn  Numerator=[0.05]  Denominator=[1 -.95]
  Out1 : Outport
  wires:
  In1/1 -> Discrete Transfer Fcn/1
  Discrete Transfer Fcn/1 -> Out1/1

== system controller_v12/signal generator/Drive_Signal3/AveragedTau_filtered ==
  note: To avoid having signal "jump",
      | we want SMOOTH transitions
      | in frequency (i.e., a weighted sum
      | of current freq and freq some delta t ago)
  note: time constant 0.002sec
      | for 10kHz samping
  In1 : Inport
  Discrete Transfer Fcn : DiscreteTransferFcn  Numerator=[0.05]  Denominator=[1 -.95]
  Out1 : Outport
  wires:
  In1/1 -> Discrete Transfer Fcn/1
  Discrete Transfer Fcn/1 -> Out1/1

== system controller_v12/signal generator/Drive_Signal3/SignalForRamp_binary ==
  note: Should output 1 or -1,
      | so signal ramps UP to 1
      | or DOWN to 0.
  In1 : Inport
  Add : Sum  Inputs=+-
  Compare To Zero : simulink/Logic and Bit Operations/Compare To Zero  relop=>  OutDataTypeStr=uint8  ZeroCross=off
  Constant : Constant
  Data Type Conversion : DataTypeConversion  OutDataTypeStr=double  SaturateOnIntegerOverflow=off  RndMeth=Floor
  Gain : Gain  Gain=2
  Out1 : Outport
  wires:
  In1/1 -> Compare To Zero/1
  Compare To Zero/1 -> Data Type Conversion/1
  Gain/1 -> Add/1
  Constant/1 -> Add/2
  Add/1 -> Out1/1
  Data Type Conversion/1 -> Gain/1

== system controller_v12/signal generator/Drive_Signal3/SignalForSin_binary ==
  note: We want this to stay "high" for 1
      | second after the actual "enable"
      | is turned off...
  In1 : Inport
  Compare To Zero : simulink/Logic and Bit Operations/Compare To Zero  relop=>  OutDataTypeStr=uint8  ZeroCross=off
  Data Type Conversion : DataTypeConversion  OutDataTypeStr=double  SaturateOnIntegerOverflow=off  RndMeth=Floor
  Out1 : Outport
  wires:
  In1/1 -> Compare To Zero/1
  Compare To Zero/1 -> Data Type Conversion/1
  Data Type Conversion/1 -> Out1/1

== system controller_v12/signal generator/Drive_Signal3/Subsystem ==
  split cycle mu : Inport
  In2 : Inport  Port=2
  1-mu : Sum  Inputs=+-
  2f : Gain  Gain=2
  2nd harmonic : Trigonometry  OutputSignalType=real
  2pi : Gain  Gain=2*pi
  Abs1 : Abs  SaturateOnIntegerOverflow=off
  Constant : Constant
  SmoothClock : DiscreteIntegrator  SampleTime=-1  ICPrevOutput=DiscIntNeverNeededParam  ICPrevScaledInput=DiscIntNeverNeededParam
  combined sines : Sum
  f : Gain
  first harmonic : Trigonometry  OutputSignalType=real
  signal with gain1 : Product  RndMeth=Zero
  signal with gain2 : Product  RndMeth=Zero
  split cycle signal : Outport
  wires:
  SmoothClock/1 -> first harmonic/1, 2f/1
  2f/1 -> 2nd harmonic/1
  2pi/1 -> SmoothClock/1
  first harmonic/1 -> signal with gain1/2
  Constant/1 -> 1-mu/1
  split cycle mu/1 -> f/1, Abs1/1
  1-mu/1 -> signal with gain1/1
  2nd harmonic/1 -> signal with gain2/2
  signal with gain1/1 -> combined sines/1
  signal with gain2/1 -> combined sines/2
  combined sines/1 -> split cycle signal/1
  In2/1 -> 2pi/1
  f/1 -> signal with gain2/1
  Abs1/1 -> 1-mu/2

== system controller_v12/signal generator/Drive_Signal4/AveragedAmp_filtered ==
  note: To avoid having signal "jump",
      | we want SMOOTH transitions
      | in frequency (i.e., a weighted sum
      | of current freq and freq some delta t ago)
  note: time constant 0.002sec
      | for 10kHz samping
  In1 : Inport
  Discrete Transfer Fcn : DiscreteTransferFcn  Numerator=[0.05]  Denominator=[1 -.95]
  Out1 : Outport
  wires:
  In1/1 -> Discrete Transfer Fcn/1
  Discrete Transfer Fcn/1 -> Out1/1

== system controller_v12/signal generator/Drive_Signal4/AveragedOffset_filtered ==
  note: To avoid having signal "jump",
      | we want SMOOTH transitions
      | in frequency (i.e., a weighted sum
      | of current freq and freq some delta t ago)
  note: c
  note: time constant 0.02sec
      | for 10kHz samping
  In1 : Inport
  Discrete Transfer Fcn : DiscreteTransferFcn  Numerator=[0.05]  Denominator=[1 -.95]
  Out1 : Outport
  wires:
  In1/1 -> Discrete Transfer Fcn/1
  Discrete Transfer Fcn/1 -> Out1/1

== system controller_v12/signal generator/Drive_Signal4/AveragedTau_filtered ==
  note: To avoid having signal "jump",
      | we want SMOOTH transitions
      | in frequency (i.e., a weighted sum
      | of current freq and freq some delta t ago)
  note: time constant 0.002sec
      | for 10kHz samping
  In1 : Inport
  Discrete Transfer Fcn : DiscreteTransferFcn  Numerator=[0.05]  Denominator=[1, -0.95]
  Out1 : Outport
  wires:
  In1/1 -> Discrete Transfer Fcn/1
  Discrete Transfer Fcn/1 -> Out1/1

== system controller_v12/signal generator/Drive_Signal4/SignalForRamp_binary ==
  note: Should output 1 or -1,
      | so signal ramps UP to 1
      | or DOWN to 0.
  In1 : Inport
  Add : Sum  Inputs=+-
  Compare To Zero : simulink/Logic and Bit Operations/Compare To Zero  relop=>  OutDataTypeStr=uint8  ZeroCross=off
  Constant : Constant
  Data Type Conversion : DataTypeConversion  OutDataTypeStr=double  SaturateOnIntegerOverflow=off  RndMeth=Floor
  Gain : Gain  Gain=2
  Out1 : Outport
  wires:
  In1/1 -> Compare To Zero/1
  Compare To Zero/1 -> Data Type Conversion/1
  Gain/1 -> Add/1
  Constant/1 -> Add/2
  Add/1 -> Out1/1
  Data Type Conversion/1 -> Gain/1

== system controller_v12/signal generator/Drive_Signal4/SignalForSin_binary ==
  note: We want this to stay "high" for 1
      | second after the actual "enable"
      | is turned off...
  In1 : Inport
  Compare To Zero : simulink/Logic and Bit Operations/Compare To Zero  relop=>  OutDataTypeStr=uint8  ZeroCross=off
  Data Type Conversion : DataTypeConversion  OutDataTypeStr=double  SaturateOnIntegerOverflow=off  RndMeth=Floor
  Out1 : Outport
  wires:
  In1/1 -> Compare To Zero/1
  Compare To Zero/1 -> Data Type Conversion/1
  Data Type Conversion/1 -> Out1/1

== system controller_v12/signal generator/Drive_Signal4/Subsystem ==
  note: positive value pushes the left wing forward
  split cycle mu : Inport
  In2 : Inport  Port=2
  1-mu : Sum  Inputs=+-
  2f : Gain  Gain=2
  2nd harmonic : Trigonometry  OutputSignalType=real
  2pi : Gain  Gain=2*pi
  Abs1 : Abs  SaturateOnIntegerOverflow=off
  Add : Sum
  Constant : Constant
  combined sines : Sum
  deg to rad : Gain  Gain=pi/180
  f : Gain  Gain=-1
  first harmonic : Trigonometry  OutputSignalType=real
  omega*t : DiscreteIntegrator  SampleTime=-1  ICPrevOutput=DiscIntNeverNeededParam  ICPrevScaledInput=DiscIntNeverNeededParam
  phase offset : Constant  Value=0
  signal with gain1 : Product  RndMeth=Zero
  signal with gain2 : Product  RndMeth=Zero
  split cycle signal : Outport
  wires:
  2f/1 -> 2nd harmonic/1
  first harmonic/1 -> signal with gain1/2
  Constant/1 -> 1-mu/1
  split cycle mu/1 -> f/1, Abs1/1
  1-mu/1 -> signal with gain1/1
  2nd harmonic/1 -> signal with gain2/2
  signal with gain1/1 -> combined sines/1
  signal with gain2/1 -> combined sines/2
  combined sines/1 -> split cycle signal/1
  f/1 -> signal with gain2/1
  Abs1/1 -> 1-mu/2
  In2/1 -> 2pi/1
  2pi/1 -> omega*t/1
  omega*t/1 -> Add/2
  Add/1 -> first harmonic/1, 2f/1
  phase offset/1 -> deg to rad/1
  deg to rad/1 -> Add/1

== system controller_v12/Adaptive Controller/adaptive system/integrator/safety2 ==
  In1 : Inport
  Compare To Constant1 : simulink/Logic and Bit Operations/Compare To Constant  relop=<=  const=inf  OutDataTypeStr=uint8
  Switch1 : Switch  Threshold=0.5  SaturateOnIntegerOverflow=off  InputSameDT=off
  zero1 : Constant  Value=0
  Out1 : Outport
  wires:
  In1/1 -> Switch1/1, Compare To Constant1/1
  Compare To Constant1/1 -> Switch1/2
  zero1/1 -> Switch1/3
  Switch1/1 -> Out1/1

== system controller_v12/Adaptive Controller/adaptive system/integrator/start ramp ==
  0.8 : Constant  Value=mdl.s_delay
  2 : Constant  Value=mdl.i_delay
  Add1 : Sum
  Add2 : Sum  Inputs=+-
  Compare To Zero : simulink/Logic and Bit Operations/Compare To Zero  relop=>  OutDataTypeStr=uint8  ZeroCross=off
  Data Type Conversion : DataTypeConversion  SaturateOnIntegerOverflow=off  RndMeth=Floor
  constant : Constant
  counter : DiscreteIntegrator  gainval=1  SampleTime=-1  UpperSaturationLimit=1  LowerSaturationLimit=0  ICPrevOutput=DiscIntNeverNeededParam  ICPrevScaledInput=DiscIntNeverNeededParam
  saturation ramp : DiscreteIntegrator  gainval=5  SampleTime=-1  LimitOutput=on  UpperSaturationLimit=1  LowerSaturationLimit=-1  ICPrevOutput=DiscIntNeverNeededParam  ICPrevScaledInput=DiscIntNeverNeededParam
  Out1 : Outport
  wires:
  constant/1 -> counter/1
  2/1 -> Add1/1
  0.8/1 -> Add1/2
  counter/1 -> Add2/1
  Add1/1 -> Add2/2
  Add2/1 -> Compare To Zero/1
  Compare To Zero/1 -> Data Type Conversion/1
  saturation ramp/1 -> Out1/1
  Data Type Conversion/1 -> saturation ramp/1

== system controller_v12/Adaptive Controller/observer/ICRA'23/Rotaion ==
  Euler : Inport
  Rotation Matrix : MATLAB Function  TreatAsAtomicUnit=on
  Rotation Matrix1 : MATLAB Function  TreatAsAtomicUnit=on
  filtered derivative : Subsystem
  R : Outport
  Rdot : Outport  Port=2
  Omega : Outport  Port=3
  wires:
  Rotation Matrix/1(R) -> filtered derivative/1(In1), Rotation Matrix1/1(R), R/1
  Euler/1 -> Rotation Matrix/1(euler_angles)
  filtered derivative/1(Out1) -> Rotation Matrix1/2(Rdot), Rdot/1
  Rotation Matrix1/1(w) -> Omega/1

== system controller_v12/Adaptive Controller/observer/ICRA'23/lateral KF observer ==
  note: x_hat_pred
  R : Inport
  f_cmd : Inport  Port=2
  xyz : Inport  Port=3
  Delay : Delay  DelayLength=1  InitialCondition=zeros(3,1)
  Delay1 : Delay  DelayLength=1  InitialCondition=zeros(3,1)  SampleTime=mdl.T
  Delay2 : Delay  DelayLength=1  InitialCondition=1
  Scope1 : Scope
  Scope2 : Scope
  Translational Dynamics & Kinamatics Lin Obs : MATLAB Function  TreatAsAtomicUnit=on
  r : Outport
  r_dot : Outport  Port=2
  r_dotdot : Outport  Port=3
  wires:
  R/1 -> Translational Dynamics & Kinamatics Lin Obs/1(R)
  Translational Dynamics & Kinamatics Lin Obs/3(acc_hat) -> r_dotdot/1
  Delay/1 -> Translational Dynamics & Kinamatics Lin Obs/5("vel_hat ")
  xyz/1 -> Translational Dynamics & Kinamatics Lin Obs/3(meas_pos)
  Translational Dynamics & Kinamatics Lin Obs/2(vel_hat) -> Scope1/1, r_dot/1, Delay/1
  Translational Dynamics & Kinamatics Lin Obs/1(pos_hat) -> Delay1/1, Scope2/1, r/1
  f_cmd/1 -> Translational Dynamics & Kinamatics Lin Obs/2(f_cmd)
  Delay1/1 -> Translational Dynamics & Kinamatics Lin Obs/4("pos_hat ")
  Translational Dynamics & Kinamatics Lin Obs/4(id_out) -> Delay2/1
  Delay2/1 -> Translational Dynamics & Kinamatics Lin Obs/6(id_in)

== system controller_v12/Adaptive Controller/observer/ICRA'23/lateral observer ==
  XYZ : Inport
  derivative filter : simulink/Discrete/Transfer Fcn Lead or Lag  PoleZ=mdl.zf1  ZeroZ=1  ICPrevOutput=0.0  ICPrevInput=0.0  DoSatur=off
      settings: SourceProductBaseCode=SL
  derivative filter1 : simulink/Discrete/Transfer Fcn Lead or Lag  PoleZ=mdl.zf2  ZeroZ=1  ICPrevOutput=0.0  ICPrevInput=0.0  DoSatur=off
      settings: SourceProductBaseCode=SL
  derivative filter2 : simulink/Discrete/Transfer Fcn Lead or Lag  PoleZ=mdl.zf2  ZeroZ=1  ICPrevOutput=0.0  ICPrevInput=0.0  DoSatur=off
      settings: SourceProductBaseCode=SL
  lat_s : Gain  Gain=mdl.f1
  lat_s2 : Gain  Gain=mdl.f2
  lat_s2_ : Gain  Gain=mdl.f2
  saturation : Subsystem
  r : Outport
  r_dot : Outport  Port=2
  r_dotdot : Outport  Port=3
  wires:
  derivative filter1/1 -> derivative filter2/1
  derivative filter/1 -> lat_s/1
  XYZ/1 -> derivative filter/1, derivative filter1/1, r/1
  derivative filter2/1 -> lat_s2/1
  lat_s/1 -> r_dot/1
  lat_s2/1 -> lat_s2_/1
  lat_s2_/1 -> saturation/1(In1)
  saturation/1(Out1) -> r_dotdot/1
